simulink model "FZ1"  (Simulink 9.3)
settings: Solver=VariableStepAuto  StartTime=0.0  StopTime=10.0  RelTol=1e-3  EnableMultiTasking=on
settings Model: Creator=Lenovo  LastModifiedBy=dell
settings DataIOCC: SaveFormat=Dataset  SignalLoggingSaveFormat=Dataset
settings DebuggingCC: UnderspecifiedInitializationDetection=Simplified  MergeDetectMultiDrivingBlocksExec=error  FcnCallInpInsideContextMsg=error  SFExecutionAtInitializationDiag=warning
settings HardwareCC: ProdBitPerPointer=64  ProdBitPerSizeT=64  ProdBitPerPtrDiffT=64  ProdLargestAtomicFloat=Float  ProdIntDivRoundTo=Zero  ProdEndianess=LittleEndian  ProdWordSize=64  ProdHWDeviceType=Intel->x86-64 (Windows64)
settings ModelReferenceCC: PropagateSignalLabelsOutOfModel=on
settings GRTTargetCC: GeneratePreprocessorConditionals=Disable all  CombineOutputUpdateFcns=on  GRTInterface=off

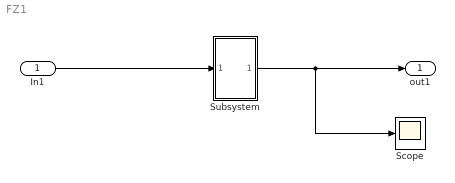
== system FZ1 ==
  In1 : Inport
  Scope : Scope
  Subsystem : Subsystem
  out1 : Outport
  wires:
  In1/1 -> Subsystem/1(In1)
  Subsystem/1(out1) -> Scope/1, out1/1

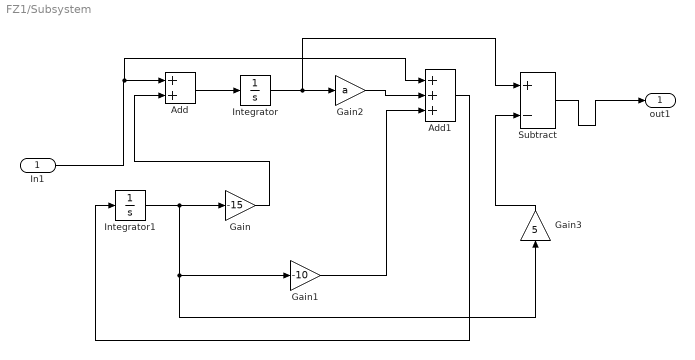
== system FZ1/Subsystem ==
  In1 : Inport
  Add : Sum
  Add1 : Sum  Inputs=+++
  Gain : Gain  Gain=-15
  Gain1 : Gain  Gain=-10
  Gain2 : Gain  Gain=a  mask{a=6}
      mask prompts: a "constant"
  Gain3 : Gain  Gain=5
  Integrator : Integrator
  Integrator1 : Integrator
  Subtract : Sum  Inputs=+-
  out1 : Outport
  wires:
  Gain3/1 -> Subtract/2
  Gain2/1 -> Add1/2
  Gain/1 -> Add/2
  Integrator1/1 -> Gain3/1, Gain1/1, Gain/1
  Gain1/1 -> Add1/3
  Add1/1 -> Integrator1/1
  In1/1 -> Add/1, Add1/1
  Integrator/1 -> Subtract/1, Gain2/1
  Add/1 -> Integrator/1
  Subtract/1 -> out1/1
